simulink model "p4_system_arch_master"  (R2020a)
settings: Solver=VariableStepAuto  StartTime=0.0  StopTime=10.0  RelTol=1e-3
(part 9 of 11)

== system p4_system_arch_master/System 5 : Enclosure and Sealing System X/5.3 Component Enclosure Peripherals X/5.3.1 Fixing, Indexation and Labeling System/5.3.1.1 Gearbox Enclosures Fixing System/5.3.1.1.20 LV connector fixing screws ==
  LV connector fixing screw 1 : ModelReference  ModelNameDialog=M6x12  SimulationMode=Normal  ModelReferenceVersion=1.1
      settings: PortSchema="{\"entries\":[{\"content\":{\"headerSize\":38,\"margin\":15,\"minimumSpacing\":25,\"sides\":[{\"content\":{\"connectorIds\":[]},\"type\":\"ConnectorPlacement.EquallySpacedRectSide\",\"uuid\":\"a1de0a4a-4383-4256-97c8-b4b7017d79c3\"},{\"content\":{\"connectorIds\":[],\"side\":\"RIGHT\"},\"type\":\"ConnectorPlacement.EquallySpacedRectSide\",\"uuid\":\"b959f0e1-b665-4773-a9ab-23b80a79bba3\"},{\"content\":{\"connectorIds\":[],\"side\":\"TOP\"},\"type\":\"ConnectorPlacement.EquallySpacedRectSide\",\"uuid\":\"884e98bd-fa8a-4556-86a7-182eb6de8f96\"}]},\"type\":\"ConnectorPlacement.EquallySpacedConnector\",\"uuid\":\"31d5ce3f-6fbe-45a5-a872-1e90bd0aea01\"}],\"packageUris\":[\"http://schema.mathworks.com/mf0/Connector/19700101\"],\"version\":\"1.0\"}"
  LV connector fixing screw 2 : ModelReference  ModelNameDialog=M6x12  SimulationMode=Normal  ModelReferenceVersion=1.1
      settings: PortSchema="{\"entries\":[{\"content\":{\"headerSize\":38,\"margin\":15,\"minimumSpacing\":25,\"sides\":[{\"content\":{\"connectorIds\":[]},\"type\":\"ConnectorPlacement.EquallySpacedRectSide\",\"uuid\":\"a1de0a4a-4383-4256-97c8-b4b7017d79c3\"},{\"content\":{\"connectorIds\":[],\"side\":\"RIGHT\"},\"type\":\"ConnectorPlacement.EquallySpacedRectSide\",\"uuid\":\"b959f0e1-b665-4773-a9ab-23b80a79bba3\"},{\"content\":{\"connectorIds\":[],\"side\":\"TOP\"},\"type\":\"ConnectorPlacement.EquallySpacedRectSide\",\"uuid\":\"884e98bd-fa8a-4556-86a7-182eb6de8f96\"}]},\"type\":\"ConnectorPlacement.EquallySpacedConnector\",\"uuid\":\"31d5ce3f-6fbe-45a5-a872-1e90bd0aea01\"}],\"packageUris\":[\"http://schema.mathworks.com/mf0/Connector/19700101\"],\"version\":\"1.0\"}"

== system p4_system_arch_master/System 5 : Enclosure and Sealing System X/5.3 Component Enclosure Peripherals X/5.3.1 Fixing, Indexation and Labeling System/5.3.1.1 Gearbox Enclosures Fixing System/5.3.1.1.21 DC connector fixing screws ==
  DC Connector Fixing Screw 1 : Subsystem
      settings: PortSchema="{\"entries\":[{\"content\":{\"headerSize\":26,\"margin\":15,\"minimumSpacing\":25,\"sides\":[{\"content\":{\"connectorIds\":[]},\"type\":\"ConnectorPlacement.EquallySpacedRectSide\",\"uuid\":\"f8ee33a9-954f-44c6-a821-b5353f3278fa\"},{\"content\":{\"connectorIds\":[],\"side\":\"RIGHT\"},\"type\":\"ConnectorPlacement.EquallySpacedRectSide\",\"uuid\":\"385f1e4f-1c89-4afc-9c19-76a078cf90bc\"},{\"content\":{\"connectorIds\":[],\"side\":\"TOP\"},\"type\":\"ConnectorPlacement.EquallySpacedRectSide\",\"uuid\":\"fc91fa49-46f5-4ba7-960e-7bda5e0416d1\"}]},\"type\":\"ConnectorPlacement.EquallySpacedConnector\",\"uuid\":\"4bf08bc6-c7ce-47fb-af04-cd9d2b5f8092\"}],\"packageUris\":[\"http://schema.mathworks.com/mf0/Connector/19700101\"],\"version\":\"1.0\"}"
  DC Connector Fixing Screw 2 : Subsystem
      settings: PortSchema="{\"entries\":[{\"content\":{\"headerSize\":26,\"margin\":15,\"minimumSpacing\":25,\"sides\":[{\"content\":{\"connectorIds\":[]},\"type\":\"ConnectorPlacement.EquallySpacedRectSide\",\"uuid\":\"f8ee33a9-954f-44c6-a821-b5353f3278fa\"},{\"content\":{\"connectorIds\":[],\"side\":\"RIGHT\"},\"type\":\"ConnectorPlacement.EquallySpacedRectSide\",\"uuid\":\"385f1e4f-1c89-4afc-9c19-76a078cf90bc\"},{\"content\":{\"connectorIds\":[],\"side\":\"TOP\"},\"type\":\"ConnectorPlacement.EquallySpacedRectSide\",\"uuid\":\"fc91fa49-46f5-4ba7-960e-7bda5e0416d1\"}]},\"type\":\"ConnectorPlacement.EquallySpacedConnector\",\"uuid\":\"4bf08bc6-c7ce-47fb-af04-cd9d2b5f8092\"}],\"packageUris\":[\"http://schema.mathworks.com/mf0/Connector/19700101\"],\"version\":\"1.0\"}"

== system p4_system_arch_master/System 5 : Enclosure and Sealing System X/5.3 Component Enclosure Peripherals X/5.3.1 Fixing, Indexation and Labeling System/5.3.1.1 Gearbox Enclosures Fixing System/5.3.1.1.25 Breather Labyrinth Cover Bolts ==

== system p4_system_arch_master/System 5 : Enclosure and Sealing System X/5.3 Component Enclosure Peripherals X/5.3.1 Fixing, Indexation and Labeling System/5.3.1.1 Gearbox Enclosures Fixing System/5.3.1.1.5 Shifting Actuator Screws ==

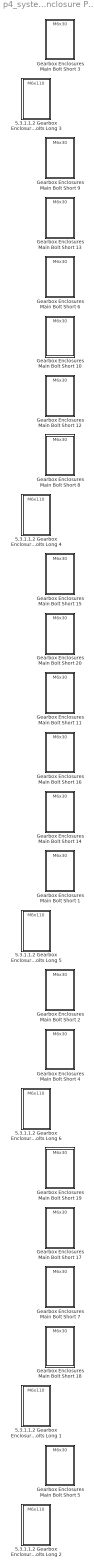
== system p4_system_arch_master/System 5 : Enclosure and Sealing System X/5.3 Component Enclosure Peripherals X/5.3.1 Fixing, Indexation and Labeling System/5.3.1.1 Gearbox Enclosures Fixing System/Gearbox Enclosure Main Bolt System ==
  5.3.1.1.2 Gearbox Enclosures Main Bolts Long {1..6} (6 alike) : ModelReference  ModelNameDialog=M6x110  SimulationMode=Normal  ModelReferenceVersion=1.1
      settings: PortSchema="{\"entries\":[{\"content\":{\"headerSize\":38,\"margin\":15,\"minimumSpacing\":25,\"sides\":[{\"content\":{\"connectorIds\":[]},\"type\":\"ConnectorPlacement.EquallySpacedRectSide\",\"uuid\":\"a1de0a4a-4383-4256-97c8-b4b7017d79c3\"},{\"content\":{\"connectorIds\":[],\"side\":\"RIGHT\"},\"type\":\"ConnectorPlacement.EquallySpacedRectSide\",\"uuid\":\"b959f0e1-b665-4773-a9ab-23b80a79bba3\"},{\"content\":{\"connectorIds\":[],\"side\":\"TOP\"},\"type\":\"ConnectorPlacement.EquallySpacedRectSide\",\"uuid\":\"884e98bd-fa8a-4556-86a7-182eb6de8f96\"}]},\"type\":\"ConnectorPlacement.EquallySpacedConnector\",\"uuid\":\"31d5ce3f-6fbe-45a5-a872-1e90bd0aea01\"}],\"packageUris\":[\"http://schema.mathworks.com/mf0/Connector/19700101\"],\"version\":\"1.0\"}"
  Gearbox Enclosures Main Bolt Short {1..20} (20 alike) : ModelReference  ModelNameDialog=M6x30  SimulationMode=Normal  ModelReferenceVersion=1.1
      settings: PortSchema="{\"entries\":[{\"content\":{\"headerSize\":38,\"margin\":15,\"minimumSpacing\":25,\"sides\":[{\"content\":{\"connectorIds\":[]},\"type\":\"ConnectorPlacement.EquallySpacedRectSide\",\"uuid\":\"a1de0a4a-4383-4256-97c8-b4b7017d79c3\"},{\"content\":{\"connectorIds\":[],\"side\":\"RIGHT\"},\"type\":\"ConnectorPlacement.EquallySpacedRectSide\",\"uuid\":\"b959f0e1-b665-4773-a9ab-23b80a79bba3\"},{\"content\":{\"connectorIds\":[],\"side\":\"TOP\"},\"type\":\"ConnectorPlacement.EquallySpacedRectSide\",\"uuid\":\"884e98bd-fa8a-4556-86a7-182eb6de8f96\"}]},\"type\":\"ConnectorPlacement.EquallySpacedConnector\",\"uuid\":\"31d5ce3f-6fbe-45a5-a872-1e90bd0aea01\"}],\"packageUris\":[\"http://schema.mathworks.com/mf0/Connector/19700101\"],\"version\":\"1.0\"}"

== system p4_system_arch_master/System 5 : Enclosure and Sealing System X/5.3 Component Enclosure Peripherals X/5.3.1 Fixing, Indexation and Labeling System/5.3.1.1 Gearbox Enclosures Fixing System/I//O Module Bolt System ==

== system p4_system_arch_master/System 5 : Enclosure and Sealing System X/5.3 Component Enclosure Peripherals X/5.3.1 Fixing, Indexation and Labeling System/5.3.1.1 Gearbox Enclosures Fixing System/Inverter fixing screws System ==
  5.3.1.1.16 Top inverter cover fixing screws : Subsystem
      settings: PortSchema="{\"entries\":[{\"content\":{\"headerSize\":26,\"margin\":15,\"minimumSpacing\":25,\"sides\":[{\"content\":{\"connectorIds\":[]},\"type\":\"ConnectorPlacement.EquallySpacedRectSide\",\"uuid\":\"f8ee33a9-954f-44c6-a821-b5353f3278fa\"},{\"content\":{\"connectorIds\":[],\"side\":\"RIGHT\"},\"type\":\"ConnectorPlacement.EquallySpacedRectSide\",\"uuid\":\"385f1e4f-1c89-4afc-9c19-76a078cf90bc\"},{\"content\":{\"connectorIds\":[],\"side\":\"TOP\"},\"type\":\"ConnectorPlacement.EquallySpacedRectSide\",\"uuid\":\"fc91fa49-46f5-4ba7-960e-7bda5e0416d1\"}]},\"type\":\"ConnectorPlacement.EquallySpacedConnector\",\"uuid\":\"4bf08bc6-c7ce-47fb-af04-cd9d2b5f8092\"}],\"packageUris\":[\"http://schema.mathworks.com/mf0/Connector/19700101\"],\"version\":\"1.0\"}"
  5.3.1.1.17 Inverter fixing screws : Subsystem
      settings: PortSchema="{\"entries\":[{\"content\":{\"headerSize\":26,\"margin\":15,\"minimumSpacing\":25,\"sides\":[{\"content\":{\"connectorIds\":[]},\"type\":\"ConnectorPlacement.EquallySpacedRectSide\",\"uuid\":\"f8ee33a9-954f-44c6-a821-b5353f3278fa\"},{\"content\":{\"connectorIds\":[],\"side\":\"RIGHT\"},\"type\":\"ConnectorPlacement.EquallySpacedRectSide\",\"uuid\":\"385f1e4f-1c89-4afc-9c19-76a078cf90bc\"},{\"content\":{\"connectorIds\":[],\"side\":\"TOP\"},\"type\":\"ConnectorPlacement.EquallySpacedRectSide\",\"uuid\":\"fc91fa49-46f5-4ba7-960e-7bda5e0416d1\"}]},\"type\":\"ConnectorPlacement.EquallySpacedConnector\",\"uuid\":\"4bf08bc6-c7ce-47fb-af04-cd9d2b5f8092\"}],\"packageUris\":[\"http://schema.mathworks.com/mf0/Connector/19700101\"],\"version\":\"1.0\"}"

== system p4_system_arch_master/System 5 : Enclosure and Sealing System X/5.3 Component Enclosure Peripherals X/5.3.1 Fixing, Indexation and Labeling System/5.3.1.1 Gearbox Enclosures Fixing System/Motorcover Securing System ==
  5.3.1.1.12 Motor cover fixing screws short : Subsystem
      settings: PortSchema="{\"entries\":[{\"content\":{\"headerSize\":26,\"margin\":15,\"minimumSpacing\":25,\"sides\":[{\"content\":{\"connectorIds\":[]},\"type\":\"ConnectorPlacement.EquallySpacedRectSide\",\"uuid\":\"f8ee33a9-954f-44c6-a821-b5353f3278fa\"},{\"content\":{\"connectorIds\":[],\"side\":\"RIGHT\"},\"type\":\"ConnectorPlacement.EquallySpacedRectSide\",\"uuid\":\"385f1e4f-1c89-4afc-9c19-76a078cf90bc\"},{\"content\":{\"connectorIds\":[],\"side\":\"TOP\"},\"type\":\"ConnectorPlacement.EquallySpacedRectSide\",\"uuid\":\"fc91fa49-46f5-4ba7-960e-7bda5e0416d1\"}]},\"type\":\"ConnectorPlacement.EquallySpacedConnector\",\"uuid\":\"4bf08bc6-c7ce-47fb-af04-cd9d2b5f8092\"}],\"packageUris\":[\"http://schema.mathworks.com/mf0/Connector/19700101\"],\"version\":\"1.0\"}"
  5.3.1.1.13 Motor cover fixing screws long : Subsystem
      settings: PortSchema="{\"entries\":[{\"content\":{\"headerSize\":26,\"margin\":15,\"minimumSpacing\":25,\"sides\":[{\"content\":{\"connectorIds\":[]},\"type\":\"ConnectorPlacement.EquallySpacedRectSide\",\"uuid\":\"f8ee33a9-954f-44c6-a821-b5353f3278fa\"},{\"content\":{\"connectorIds\":[],\"side\":\"RIGHT\"},\"type\":\"ConnectorPlacement.EquallySpacedRectSide\",\"uuid\":\"385f1e4f-1c89-4afc-9c19-76a078cf90bc\"},{\"content\":{\"connectorIds\":[],\"side\":\"TOP\"},\"type\":\"ConnectorPlacement.EquallySpacedRectSide\",\"uuid\":\"fc91fa49-46f5-4ba7-960e-7bda5e0416d1\"}]},\"type\":\"ConnectorPlacement.EquallySpacedConnector\",\"uuid\":\"4bf08bc6-c7ce-47fb-af04-cd9d2b5f8092\"}],\"packageUris\":[\"http://schema.mathworks.com/mf0/Connector/19700101\"],\"version\":\"1.0\"}"

== system p4_system_arch_master/System 5 : Enclosure and Sealing System X/5.3 Component Enclosure Peripherals X/5.3.1 Fixing, Indexation and Labeling System/5.3.1.1 Gearbox Enclosures Fixing System/Oil Baffle securing System ==
  5.3.1.1.19 Oil baffle RH bolts : Subsystem
      settings: PortSchema="{\"entries\":[{\"content\":{\"headerSize\":26,\"margin\":15,\"minimumSpacing\":25,\"sides\":[{\"content\":{\"connectorIds\":[]},\"type\":\"ConnectorPlacement.EquallySpacedRectSide\",\"uuid\":\"f8ee33a9-954f-44c6-a821-b5353f3278fa\"},{\"content\":{\"connectorIds\":[],\"side\":\"RIGHT\"},\"type\":\"ConnectorPlacement.EquallySpacedRectSide\",\"uuid\":\"385f1e4f-1c89-4afc-9c19-76a078cf90bc\"},{\"content\":{\"connectorIds\":[],\"side\":\"TOP\"},\"type\":\"ConnectorPlacement.EquallySpacedRectSide\",\"uuid\":\"fc91fa49-46f5-4ba7-960e-7bda5e0416d1\"}]},\"type\":\"ConnectorPlacement.EquallySpacedConnector\",\"uuid\":\"4bf08bc6-c7ce-47fb-af04-cd9d2b5f8092\"}],\"packageUris\":[\"http://schema.mathworks.com/mf0/Connector/19700101\"],\"version\":\"1.0\"}"
  "5.3.1.1.9 Rear Oil Baffle LH Bolts " : Subsystem
      settings: PortSchema="{\"entries\":[{\"content\":{\"headerSize\":26,\"margin\":15,\"minimumSpacing\":25,\"sides\":[{\"content\":{\"connectorIds\":[]},\"type\":\"ConnectorPlacement.EquallySpacedRectSide\",\"uuid\":\"f8ee33a9-954f-44c6-a821-b5353f3278fa\"},{\"content\":{\"connectorIds\":[],\"side\":\"RIGHT\"},\"type\":\"ConnectorPlacement.EquallySpacedRectSide\",\"uuid\":\"385f1e4f-1c89-4afc-9c19-76a078cf90bc\"},{\"content\":{\"connectorIds\":[],\"side\":\"TOP\"},\"type\":\"ConnectorPlacement.EquallySpacedRectSide\",\"uuid\":\"fc91fa49-46f5-4ba7-960e-7bda5e0416d1\"}]},\"type\":\"ConnectorPlacement.EquallySpacedConnector\",\"uuid\":\"4bf08bc6-c7ce-47fb-af04-cd9d2b5f8092\"}],\"packageUris\":[\"http://schema.mathworks.com/mf0/Connector/19700101\"],\"version\":\"1.0\"}"

== system p4_system_arch_master/System 5 : Enclosure and Sealing System X/5.3 Component Enclosure Peripherals X/5.3.1 Fixing, Indexation and Labeling System/5.3.1.1 Gearbox Enclosures Fixing System/Oil Catcher Bolts System ==
  5.3.1.1.7 Oil Catcher B3 Bolts : Subsystem
      settings: PortSchema="{\"entries\":[{\"content\":{\"headerSize\":26,\"margin\":15,\"minimumSpacing\":25,\"sides\":[{\"content\":{\"connectorIds\":[]},\"type\":\"ConnectorPlacement.EquallySpacedRectSide\",\"uuid\":\"f8ee33a9-954f-44c6-a821-b5353f3278fa\"},{\"content\":{\"connectorIds\":[],\"side\":\"RIGHT\"},\"type\":\"ConnectorPlacement.EquallySpacedRectSide\",\"uuid\":\"385f1e4f-1c89-4afc-9c19-76a078cf90bc\"},{\"content\":{\"connectorIds\":[],\"side\":\"TOP\"},\"type\":\"ConnectorPlacement.EquallySpacedRectSide\",\"uuid\":\"fc91fa49-46f5-4ba7-960e-7bda5e0416d1\"}]},\"type\":\"ConnectorPlacement.EquallySpacedConnector\",\"uuid\":\"4bf08bc6-c7ce-47fb-af04-cd9d2b5f8092\"}],\"packageUris\":[\"http://schema.mathworks.com/mf0/Connector/19700101\"],\"version\":\"1.0\"}"
  5.3.1.1.8 Oil Catcher B1 Bolts : Subsystem
      settings: PortSchema="{\"entries\":[{\"content\":{\"headerSize\":26,\"margin\":15,\"minimumSpacing\":25,\"sides\":[{\"content\":{\"connectorIds\":[]},\"type\":\"ConnectorPlacement.EquallySpacedRectSide\",\"uuid\":\"f8ee33a9-954f-44c6-a821-b5353f3278fa\"},{\"content\":{\"connectorIds\":[],\"side\":\"RIGHT\"},\"type\":\"ConnectorPlacement.EquallySpacedRectSide\",\"uuid\":\"385f1e4f-1c89-4afc-9c19-76a078cf90bc\"},{\"content\":{\"connectorIds\":[],\"side\":\"TOP\"},\"type\":\"ConnectorPlacement.EquallySpacedRectSide\",\"uuid\":\"fc91fa49-46f5-4ba7-960e-7bda5e0416d1\"}]},\"type\":\"ConnectorPlacement.EquallySpacedConnector\",\"uuid\":\"4bf08bc6-c7ce-47fb-af04-cd9d2b5f8092\"}],\"packageUris\":[\"http://schema.mathworks.com/mf0/Connector/19700101\"],\"version\":\"1.0\"}"

== system p4_system_arch_master/System 5 : Enclosure and Sealing System X/5.3 Component Enclosure Peripherals X/5.3.1 Fixing, Indexation and Labeling System/5.3.1.1 Gearbox Enclosures Fixing System/Resolver System ==
  5.3.1.1.14 Resolver fixing screws : Subsystem
      settings: PortSchema="{\"entries\":[{\"content\":{\"headerSize\":26,\"margin\":15,\"minimumSpacing\":25,\"sides\":[{\"content\":{\"connectorIds\":[]},\"type\":\"ConnectorPlacement.EquallySpacedRectSide\",\"uuid\":\"f8ee33a9-954f-44c6-a821-b5353f3278fa\"},{\"content\":{\"connectorIds\":[],\"side\":\"RIGHT\"},\"type\":\"ConnectorPlacement.EquallySpacedRectSide\",\"uuid\":\"385f1e4f-1c89-4afc-9c19-76a078cf90bc\"},{\"content\":{\"connectorIds\":[],\"side\":\"TOP\"},\"type\":\"ConnectorPlacement.EquallySpacedRectSide\",\"uuid\":\"fc91fa49-46f5-4ba7-960e-7bda5e0416d1\"}]},\"type\":\"ConnectorPlacement.EquallySpacedConnector\",\"uuid\":\"4bf08bc6-c7ce-47fb-af04-cd9d2b5f8092\"}],\"packageUris\":[\"http://schema.mathworks.com/mf0/Connector/19700101\"],\"version\":\"1.0\"}"
  5.3.1.1.15 Resolver cover fixing screws : Subsystem
      settings: PortSchema="{\"entries\":[{\"content\":{\"headerSize\":26,\"margin\":15,\"minimumSpacing\":25,\"sides\":[{\"content\":{\"connectorIds\":[]},\"type\":\"ConnectorPlacement.EquallySpacedRectSide\",\"uuid\":\"f8ee33a9-954f-44c6-a821-b5353f3278fa\"},{\"content\":{\"connectorIds\":[],\"side\":\"RIGHT\"},\"type\":\"ConnectorPlacement.EquallySpacedRectSide\",\"uuid\":\"385f1e4f-1c89-4afc-9c19-76a078cf90bc\"},{\"content\":{\"connectorIds\":[],\"side\":\"TOP\"},\"type\":\"ConnectorPlacement.EquallySpacedRectSide\",\"uuid\":\"fc91fa49-46f5-4ba7-960e-7bda5e0416d1\"}]},\"type\":\"ConnectorPlacement.EquallySpacedConnector\",\"uuid\":\"4bf08bc6-c7ce-47fb-af04-cd9d2b5f8092\"}],\"packageUris\":[\"http://schema.mathworks.com/mf0/Connector/19700101\"],\"version\":\"1.0\"}"
  5.3.1.1.24 Resolver Plate : Subsystem
      settings: PortSchema="{\"entries\":[{\"content\":{\"headerSize\":26,\"margin\":15,\"minimumSpacing\":25,\"sides\":[{\"content\":{\"connectorIds\":[]},\"type\":\"ConnectorPlacement.EquallySpacedRectSide\",\"uuid\":\"f8ee33a9-954f-44c6-a821-b5353f3278fa\"},{\"content\":{\"connectorIds\":[],\"side\":\"RIGHT\"},\"type\":\"ConnectorPlacement.EquallySpacedRectSide\",\"uuid\":\"385f1e4f-1c89-4afc-9c19-76a078cf90bc\"},{\"content\":{\"connectorIds\":[],\"side\":\"TOP\"},\"type\":\"ConnectorPlacement.EquallySpacedRectSide\",\"uuid\":\"fc91fa49-46f5-4ba7-960e-7bda5e0416d1\"}]},\"type\":\"ConnectorPlacement.EquallySpacedConnector\",\"uuid\":\"4bf08bc6-c7ce-47fb-af04-cd9d2b5f8092\"}],\"packageUris\":[\"http://schema.mathworks.com/mf0/Connector/19700101\"],\"version\":\"1.0\"}"

== system p4_system_arch_master/System 5 : Enclosure and Sealing System X/5.3 Component Enclosure Peripherals X/5.3.1 Fixing, Indexation and Labeling System/5.3.1.1 Gearbox Enclosures Fixing System/Shifting Angle Sensor Bolts System ==
  5.3.1.1.23 Shifting Angle Sensor Bolts : Subsystem
      settings: PortSchema="{\"entries\":[{\"content\":{\"headerSize\":26,\"margin\":15,\"minimumSpacing\":25,\"sides\":[{\"content\":{\"connectorIds\":[]},\"type\":\"ConnectorPlacement.EquallySpacedRectSide\",\"uuid\":\"f8ee33a9-954f-44c6-a821-b5353f3278fa\"},{\"content\":{\"connectorIds\":[],\"side\":\"RIGHT\"},\"type\":\"ConnectorPlacement.EquallySpacedRectSide\",\"uuid\":\"385f1e4f-1c89-4afc-9c19-76a078cf90bc\"},{\"content\":{\"connectorIds\":[],\"side\":\"TOP\"},\"type\":\"ConnectorPlacement.EquallySpacedRectSide\",\"uuid\":\"fc91fa49-46f5-4ba7-960e-7bda5e0416d1\"}]},\"type\":\"ConnectorPlacement.EquallySpacedConnector\",\"uuid\":\"4bf08bc6-c7ce-47fb-af04-cd9d2b5f8092\"}],\"packageUris\":[\"http://schema.mathworks.com/mf0/Connector/19700101\"],\"version\":\"1.0\"}"

== system p4_system_arch_master/System 5 : Enclosure and Sealing System X/5.3 Component Enclosure Peripherals X/5.3.1 Fixing, Indexation and Labeling System/5.3.1.1 Gearbox Enclosures Fixing System/Shifting Cover Bolts System ==
  5.3.1.1.4 Shifting Cover Bolt 1 : Subsystem
      settings: PortSchema="{\"entries\":[{\"content\":{\"headerSize\":26,\"margin\":15,\"minimumSpacing\":25,\"sides\":[{\"content\":{\"connectorIds\":[]},\"type\":\"ConnectorPlacement.EquallySpacedRectSide\",\"uuid\":\"f8ee33a9-954f-44c6-a821-b5353f3278fa\"},{\"content\":{\"connectorIds\":[],\"side\":\"RIGHT\"},\"type\":\"ConnectorPlacement.EquallySpacedRectSide\",\"uuid\":\"385f1e4f-1c89-4afc-9c19-76a078cf90bc\"},{\"content\":{\"connectorIds\":[],\"side\":\"TOP\"},\"type\":\"ConnectorPlacement.EquallySpacedRectSide\",\"uuid\":\"fc91fa49-46f5-4ba7-960e-7bda5e0416d1\"}]},\"type\":\"ConnectorPlacement.EquallySpacedConnector\",\"uuid\":\"4bf08bc6-c7ce-47fb-af04-cd9d2b5f8092\"}],\"packageUris\":[\"http://schema.mathworks.com/mf0/Connector/19700101\"],\"version\":\"1.0\"}"
  5.3.1.1.4 Shifting Cover Bolt 2 : Subsystem
      settings: PortSchema="{\"entries\":[{\"content\":{\"headerSize\":26,\"margin\":15,\"minimumSpacing\":25,\"sides\":[{\"content\":{\"connectorIds\":[]},\"type\":\"ConnectorPlacement.EquallySpacedRectSide\",\"uuid\":\"f8ee33a9-954f-44c6-a821-b5353f3278fa\"},{\"content\":{\"connectorIds\":[],\"side\":\"RIGHT\"},\"type\":\"ConnectorPlacement.EquallySpacedRectSide\",\"uuid\":\"385f1e4f-1c89-4afc-9c19-76a078cf90bc\"},{\"content\":{\"connectorIds\":[],\"side\":\"TOP\"},\"type\":\"ConnectorPlacement.EquallySpacedRectSide\",\"uuid\":\"fc91fa49-46f5-4ba7-960e-7bda5e0416d1\"}]},\"type\":\"ConnectorPlacement.EquallySpacedConnector\",\"uuid\":\"4bf08bc6-c7ce-47fb-af04-cd9d2b5f8092\"}],\"packageUris\":[\"http://schema.mathworks.com/mf0/Connector/19700101\"],\"version\":\"1.0\"}"
  5.3.1.1.4 Shifting Cover Bolt 3 : Subsystem
      settings: PortSchema="{\"entries\":[{\"content\":{\"headerSize\":26,\"margin\":15,\"minimumSpacing\":25,\"sides\":[{\"content\":{\"connectorIds\":[]},\"type\":\"ConnectorPlacement.EquallySpacedRectSide\",\"uuid\":\"f8ee33a9-954f-44c6-a821-b5353f3278fa\"},{\"content\":{\"connectorIds\":[],\"side\":\"RIGHT\"},\"type\":\"ConnectorPlacement.EquallySpacedRectSide\",\"uuid\":\"385f1e4f-1c89-4afc-9c19-76a078cf90bc\"},{\"content\":{\"connectorIds\":[],\"side\":\"TOP\"},\"type\":\"ConnectorPlacement.EquallySpacedRectSide\",\"uuid\":\"fc91fa49-46f5-4ba7-960e-7bda5e0416d1\"}]},\"type\":\"ConnectorPlacement.EquallySpacedConnector\",\"uuid\":\"4bf08bc6-c7ce-47fb-af04-cd9d2b5f8092\"}],\"packageUris\":[\"http://schema.mathworks.com/mf0/Connector/19700101\"],\"version\":\"1.0\"}"
  5.3.1.1.4 Shifting Cover Bolt 4 : Subsystem
      settings: PortSchema="{\"entries\":[{\"content\":{\"headerSize\":26,\"margin\":15,\"minimumSpacing\":25,\"sides\":[{\"content\":{\"connectorIds\":[]},\"type\":\"ConnectorPlacement.EquallySpacedRectSide\",\"uuid\":\"f8ee33a9-954f-44c6-a821-b5353f3278fa\"},{\"content\":{\"connectorIds\":[],\"side\":\"RIGHT\"},\"type\":\"ConnectorPlacement.EquallySpacedRectSide\",\"uuid\":\"385f1e4f-1c89-4afc-9c19-76a078cf90bc\"},{\"content\":{\"connectorIds\":[],\"side\":\"TOP\"},\"type\":\"ConnectorPlacement.EquallySpacedRectSide\",\"uuid\":\"fc91fa49-46f5-4ba7-960e-7bda5e0416d1\"}]},\"type\":\"ConnectorPlacement.EquallySpacedConnector\",\"uuid\":\"4bf08bc6-c7ce-47fb-af04-cd9d2b5f8092\"}],\"packageUris\":[\"http://schema.mathworks.com/mf0/Connector/19700101\"],\"version\":\"1.0\"}"

== system p4_system_arch_master/System 5 : Enclosure and Sealing System X/5.3 Component Enclosure Peripherals X/5.3.1 Fixing, Indexation and Labeling System/5.3.1.1 Gearbox Enclosures Fixing System/Speed Sensor Bolt System ==
  5.3.1.1.6 Speed Sensor LH Bolt : ModelReference  ModelNameDialog=M6x14  SimulationMode=Normal  ModelReferenceVersion=1.1
      settings: PortSchema="{\"entries\":[{\"content\":{\"headerSize\":38,\"margin\":15,\"minimumSpacing\":25,\"sides\":[{\"content\":{\"connectorIds\":[]},\"type\":\"ConnectorPlacement.EquallySpacedRectSide\",\"uuid\":\"a1de0a4a-4383-4256-97c8-b4b7017d79c3\"},{\"content\":{\"connectorIds\":[],\"side\":\"RIGHT\"},\"type\":\"ConnectorPlacement.EquallySpacedRectSide\",\"uuid\":\"b959f0e1-b665-4773-a9ab-23b80a79bba3\"},{\"content\":{\"connectorIds\":[],\"side\":\"TOP\"},\"type\":\"ConnectorPlacement.EquallySpacedRectSide\",\"uuid\":\"884e98bd-fa8a-4556-86a7-182eb6de8f96\"}]},\"type\":\"ConnectorPlacement.EquallySpacedConnector\",\"uuid\":\"31d5ce3f-6fbe-45a5-a872-1e90bd0aea01\"}],\"packageUris\":[\"http://schema.mathworks.com/mf0/Connector/19700101\"],\"version\":\"1.0\"}"
  5.3.1.1.6 Speed Sensor RH Bolt : ModelReference  ModelNameDialog=M6x14  SimulationMode=Normal  ModelReferenceVersion=1.1
      settings: PortSchema="{\"entries\":[{\"content\":{\"headerSize\":38,\"margin\":15,\"minimumSpacing\":25,\"sides\":[{\"content\":{\"connectorIds\":[]},\"type\":\"ConnectorPlacement.EquallySpacedRectSide\",\"uuid\":\"a1de0a4a-4383-4256-97c8-b4b7017d79c3\"},{\"content\":{\"connectorIds\":[],\"side\":\"RIGHT\"},\"type\":\"ConnectorPlacement.EquallySpacedRectSide\",\"uuid\":\"b959f0e1-b665-4773-a9ab-23b80a79bba3\"},{\"content\":{\"connectorIds\":[],\"side\":\"TOP\"},\"type\":\"ConnectorPlacement.EquallySpacedRectSide\",\"uuid\":\"884e98bd-fa8a-4556-86a7-182eb6de8f96\"}]},\"type\":\"ConnectorPlacement.EquallySpacedConnector\",\"uuid\":\"31d5ce3f-6fbe-45a5-a872-1e90bd0aea01\"}],\"packageUris\":[\"http://schema.mathworks.com/mf0/Connector/19700101\"],\"version\":\"1.0\"}"

== system p4_system_arch_master/System 5 : Enclosure and Sealing System X/5.3 Component Enclosure Peripherals X/5.3.1 Fixing, Indexation and Labeling System/5.3.1.1 Gearbox Enclosures Fixing System/Stator Securing System ==
  5.3.1.1.10 Stator bolt {1..4} (4 alike) : ModelReference  ModelNameDialog=M8x220  SimulationMode=Normal  ModelReferenceVersion=1.1
      settings: PortSchema="{\"entries\":[{\"content\":{\"headerSize\":38,\"margin\":15,\"minimumSpacing\":25,\"sides\":[{\"content\":{\"connectorIds\":[]},\"type\":\"ConnectorPlacement.EquallySpacedRectSide\",\"uuid\":\"a1de0a4a-4383-4256-97c8-b4b7017d79c3\"},{\"content\":{\"connectorIds\":[],\"side\":\"RIGHT\"},\"type\":\"ConnectorPlacement.EquallySpacedRectSide\",\"uuid\":\"b959f0e1-b665-4773-a9ab-23b80a79bba3\"},{\"content\":{\"connectorIds\":[],\"side\":\"TOP\"},\"type\":\"ConnectorPlacement.EquallySpacedRectSide\",\"uuid\":\"884e98bd-fa8a-4556-86a7-182eb6de8f96\"}]},\"type\":\"ConnectorPlacement.EquallySpacedConnector\",\"uuid\":\"31d5ce3f-6fbe-45a5-a872-1e90bd0aea01\"}],\"packageUris\":[\"http://schema.mathworks.com/mf0/Connector/19700101\"],\"version\":\"1.0\"}"
  5.3.1.1.11 Stator piston bush (sleeves) {1..4} (4 alike) : ModelReference  ModelNameDialog=StatorPistonBushSleeves  SimulationMode=Normal  ModelReferenceVersion=1.2
      settings: PortSchema="{\"entries\":[{\"content\":{\"headerSize\":38,\"margin\":15,\"minimumSpacing\":25,\"sides\":[{\"content\":{\"connectorIds\":[]},\"type\":\"ConnectorPlacement.EquallySpacedRectSide\",\"uuid\":\"a1de0a4a-4383-4256-97c8-b4b7017d79c3\"},{\"content\":{\"connectorIds\":[],\"side\":\"RIGHT\"},\"type\":\"ConnectorPlacement.EquallySpacedRectSide\",\"uuid\":\"b959f0e1-b665-4773-a9ab-23b80a79bba3\"},{\"content\":{\"connectorIds\":[],\"side\":\"TOP\"},\"type\":\"ConnectorPlacement.EquallySpacedRectSide\",\"uuid\":\"884e98bd-fa8a-4556-86a7-182eb6de8f96\"}]},\"type\":\"ConnectorPlacement.EquallySpacedConnector\",\"uuid\":\"31d5ce3f-6fbe-45a5-a872-1e90bd0aea01\"}],\"packageUris\":[\"http://schema.mathworks.com/mf0/Connector/19700101\"],\"version\":\"1.0\"}"

== system p4_system_arch_master/System 5 : Enclosure and Sealing System X/5.3 Component Enclosure Peripherals X/5.3.2 Lubrication and Cooling Peripherals/5.3.2.1 Lubrication System Peripherals/5.3.2.1.1 Oil filling plug ==

== system p4_system_arch_master/System 5 : Enclosure and Sealing System X/5.3 Component Enclosure Peripherals X/5.3.2 Lubrication and Cooling Peripherals/5.3.2.1 Lubrication System Peripherals/5.3.2.1.2 Oil Catcher B1 ==

== system p4_system_arch_master/System 5 : Enclosure and Sealing System X/5.3 Component Enclosure Peripherals X/5.3.2 Lubrication and Cooling Peripherals/5.3.2.1 Lubrication System Peripherals/5.3.2.1.3 Oil Catcher B3 ==

== system p4_system_arch_master/System 5 : Enclosure and Sealing System X/5.3 Component Enclosure Peripherals X/5.3.2 Lubrication and Cooling Peripherals/5.3.2.1 Lubrication System Peripherals/5.3.2.1.4 Rear Oil Baffle LH ==

== system p4_system_arch_master/System 5 : Enclosure and Sealing System X/5.3 Component Enclosure Peripherals X/5.3.2 Lubrication and Cooling Peripherals/5.3.2.1 Lubrication System Peripherals/5.3.2.1.5 Oil drain plug ==

== system p4_system_arch_master/System 5 : Enclosure and Sealing System X/5.3 Component Enclosure Peripherals X/5.3.2 Lubrication and Cooling Peripherals/5.3.2.1 Lubrication System Peripherals/5.3.2.1.6 Rear Oil Baffle RH ==

== system p4_system_arch_master/System 5 : Enclosure and Sealing System X/5.3 Component Enclosure Peripherals X/5.3.2 Lubrication and Cooling Peripherals/5.3.2.1 Lubrication System Peripherals/5.3.2.1.7 Breather Labyrinth Cover ==

== system p4_system_arch_master/System 5 : Enclosure and Sealing System X/5.3 Component Enclosure Peripherals X/5.3.2 Lubrication and Cooling Peripherals/5.3.2.1 Lubrication System Peripherals/5.3.2.1.8 Oil Disc B3 ==

== system p4_system_arch_master/System 5 : Enclosure and Sealing System X/5.3 Component Enclosure Peripherals X/5.3.2 Lubrication and Cooling Peripherals/5.3.2.3 Gearbox Venting & Aerating System/5.3.2.3.1 Breather ==

== system p4_system_arch_master/System 6 : Sensor and Actuation System/6.1 Sensor System /6.1.4 Gear Selection Position Measurement SubSystem /6.1.4.1 Drum Angular Position Measurement Sensor SubSystem /6.1.4.1.1 Drum Angular Position measurement sensor subsystem - body  ==

== system p4_system_arch_master/System 6 : Sensor and Actuation System/6.1 Sensor System /6.1.4 Gear Selection Position Measurement SubSystem /6.1.4.1 Drum Angular Position Measurement Sensor SubSystem /6.1.4.1.2 Drum Angular Position Measurement Sensor Wires  ==
  Wire 1 : Subsystem
      settings: PortSchema="{\"entries\":[{\"content\":{\"headerSize\":26,\"margin\":15,\"minimumSpacing\":25,\"sides\":[{\"content\":{\"connectorIds\":[]},\"type\":\"ConnectorPlacement.EquallySpacedRectSide\",\"uuid\":\"f8ee33a9-954f-44c6-a821-b5353f3278fa\"},{\"content\":{\"connectorIds\":[],\"side\":\"RIGHT\"},\"type\":\"ConnectorPlacement.EquallySpacedRectSide\",\"uuid\":\"385f1e4f-1c89-4afc-9c19-76a078cf90bc\"},{\"content\":{\"connectorIds\":[],\"side\":\"TOP\"},\"type\":\"ConnectorPlacement.EquallySpacedRectSide\",\"uuid\":\"fc91fa49-46f5-4ba7-960e-7bda5e0416d1\"}]},\"type\":\"ConnectorPlacement.EquallySpacedConnector\",\"uuid\":\"4bf08bc6-c7ce-47fb-af04-cd9d2b5f8092\"}],\"packageUris\":[\"http://schema.mathworks.com/mf0/Connector/19700101\"],\"version\":\"1.0\"}"
  Wire 2 : Subsystem
      settings: PortSchema="{\"entries\":[{\"content\":{\"headerSize\":26,\"margin\":15,\"minimumSpacing\":25,\"sides\":[{\"content\":{\"connectorIds\":[]},\"type\":\"ConnectorPlacement.EquallySpacedRectSide\",\"uuid\":\"f8ee33a9-954f-44c6-a821-b5353f3278fa\"},{\"content\":{\"connectorIds\":[],\"side\":\"RIGHT\"},\"type\":\"ConnectorPlacement.EquallySpacedRectSide\",\"uuid\":\"385f1e4f-1c89-4afc-9c19-76a078cf90bc\"},{\"content\":{\"connectorIds\":[],\"side\":\"TOP\"},\"type\":\"ConnectorPlacement.EquallySpacedRectSide\",\"uuid\":\"fc91fa49-46f5-4ba7-960e-7bda5e0416d1\"}]},\"type\":\"ConnectorPlacement.EquallySpacedConnector\",\"uuid\":\"4bf08bc6-c7ce-47fb-af04-cd9d2b5f8092\"}],\"packageUris\":[\"http://schema.mathworks.com/mf0/Connector/19700101\"],\"version\":\"1.0\"}"
  Wire 3 : Subsystem
      settings: PortSchema="{\"entries\":[{\"content\":{\"headerSize\":26,\"margin\":15,\"minimumSpacing\":25,\"sides\":[{\"content\":{\"connectorIds\":[]},\"type\":\"ConnectorPlacement.EquallySpacedRectSide\",\"uuid\":\"f8ee33a9-954f-44c6-a821-b5353f3278fa\"},{\"content\":{\"connectorIds\":[],\"side\":\"RIGHT\"},\"type\":\"ConnectorPlacement.EquallySpacedRectSide\",\"uuid\":\"385f1e4f-1c89-4afc-9c19-76a078cf90bc\"},{\"content\":{\"connectorIds\":[],\"side\":\"TOP\"},\"type\":\"ConnectorPlacement.EquallySpacedRectSide\",\"uuid\":\"fc91fa49-46f5-4ba7-960e-7bda5e0416d1\"}]},\"type\":\"ConnectorPlacement.EquallySpacedConnector\",\"uuid\":\"4bf08bc6-c7ce-47fb-af04-cd9d2b5f8092\"}],\"packageUris\":[\"http://schema.mathworks.com/mf0/Connector/19700101\"],\"version\":\"1.0\"}"
  Wire 4 : Subsystem
      settings: PortSchema="{\"entries\":[{\"content\":{\"headerSize\":26,\"margin\":15,\"minimumSpacing\":25,\"sides\":[{\"content\":{\"connectorIds\":[]},\"type\":\"ConnectorPlacement.EquallySpacedRectSide\",\"uuid\":\"f8ee33a9-954f-44c6-a821-b5353f3278fa\"},{\"content\":{\"connectorIds\":[],\"side\":\"RIGHT\"},\"type\":\"ConnectorPlacement.EquallySpacedRectSide\",\"uuid\":\"385f1e4f-1c89-4afc-9c19-76a078cf90bc\"},{\"content\":{\"connectorIds\":[],\"side\":\"TOP\"},\"type\":\"ConnectorPlacement.EquallySpacedRectSide\",\"uuid\":\"fc91fa49-46f5-4ba7-960e-7bda5e0416d1\"}]},\"type\":\"ConnectorPlacement.EquallySpacedConnector\",\"uuid\":\"4bf08bc6-c7ce-47fb-af04-cd9d2b5f8092\"}],\"packageUris\":[\"http://schema.mathworks.com/mf0/Connector/19700101\"],\"version\":\"1.0\"}"

== system p4_system_arch_master/System 6 : Sensor and Actuation System/6.1 Sensor System /6.1.4 Gear Selection Position Measurement SubSystem /6.1.4.2 Drum Angular Position Measurement Magnet SubSystem /6.1.4.2.1 Drum Angular position Measurement magent subsystem - body  ==

== system p4_system_arch_master/System 6 : Sensor and Actuation System/6.1 Sensor System /6.1.7 Motor Position Measurement Subsystem /6.1.7.1 Motor Resolver - Stator Subsystem /6.1.7.1.1 Motor Resolver Stator Subsystem - Body ==

== system p4_system_arch_master/System 6 : Sensor and Actuation System/6.1 Sensor System /6.1.7 Motor Position Measurement Subsystem /6.1.7.1 Motor Resolver - Stator Subsystem /6.1.7.1.2 Motor Resolver Stator Subsystem Wires ==
  Wire 1 : Subsystem
      settings: PortSchema="{\"entries\":[{\"content\":{\"headerSize\":26,\"margin\":15,\"minimumSpacing\":25,\"sides\":[{\"content\":{\"connectorIds\":[]},\"type\":\"ConnectorPlacement.EquallySpacedRectSide\",\"uuid\":\"f8ee33a9-954f-44c6-a821-b5353f3278fa\"},{\"content\":{\"connectorIds\":[],\"side\":\"RIGHT\"},\"type\":\"ConnectorPlacement.EquallySpacedRectSide\",\"uuid\":\"385f1e4f-1c89-4afc-9c19-76a078cf90bc\"},{\"content\":{\"connectorIds\":[],\"side\":\"TOP\"},\"type\":\"ConnectorPlacement.EquallySpacedRectSide\",\"uuid\":\"fc91fa49-46f5-4ba7-960e-7bda5e0416d1\"}]},\"type\":\"ConnectorPlacement.EquallySpacedConnector\",\"uuid\":\"4bf08bc6-c7ce-47fb-af04-cd9d2b5f8092\"}],\"packageUris\":[\"http://schema.mathworks.com/mf0/Connector/19700101\"],\"version\":\"1.0\"}"
  Wire 2 : Subsystem
      settings: PortSchema="{\"entries\":[{\"content\":{\"headerSize\":26,\"margin\":15,\"minimumSpacing\":25,\"sides\":[{\"content\":{\"connectorIds\":[]},\"type\":\"ConnectorPlacement.EquallySpacedRectSide\",\"uuid\":\"f8ee33a9-954f-44c6-a821-b5353f3278fa\"},{\"content\":{\"connectorIds\":[],\"side\":\"RIGHT\"},\"type\":\"ConnectorPlacement.EquallySpacedRectSide\",\"uuid\":\"385f1e4f-1c89-4afc-9c19-76a078cf90bc\"},{\"content\":{\"connectorIds\":[],\"side\":\"TOP\"},\"type\":\"ConnectorPlacement.EquallySpacedRectSide\",\"uuid\":\"fc91fa49-46f5-4ba7-960e-7bda5e0416d1\"}]},\"type\":\"ConnectorPlacement.EquallySpacedConnector\",\"uuid\":\"4bf08bc6-c7ce-47fb-af04-cd9d2b5f8092\"}],\"packageUris\":[\"http://schema.mathworks.com/mf0/Connector/19700101\"],\"version\":\"1.0\"}"
  Wire 3 : Subsystem
      settings: PortSchema="{\"entries\":[{\"content\":{\"headerSize\":26,\"margin\":15,\"minimumSpacing\":25,\"sides\":[{\"content\":{\"connectorIds\":[]},\"type\":\"ConnectorPlacement.EquallySpacedRectSide\",\"uuid\":\"f8ee33a9-954f-44c6-a821-b5353f3278fa\"},{\"content\":{\"connectorIds\":[],\"side\":\"RIGHT\"},\"type\":\"ConnectorPlacement.EquallySpacedRectSide\",\"uuid\":\"385f1e4f-1c89-4afc-9c19-76a078cf90bc\"},{\"content\":{\"connectorIds\":[],\"side\":\"TOP\"},\"type\":\"ConnectorPlacement.EquallySpacedRectSide\",\"uuid\":\"fc91fa49-46f5-4ba7-960e-7bda5e0416d1\"}]},\"type\":\"ConnectorPlacement.EquallySpacedConnector\",\"uuid\":\"4bf08bc6-c7ce-47fb-af04-cd9d2b5f8092\"}],\"packageUris\":[\"http://schema.mathworks.com/mf0/Connector/19700101\"],\"version\":\"1.0\"}"
  Wire 4 : Subsystem
      settings: PortSchema="{\"entries\":[{\"content\":{\"headerSize\":26,\"margin\":15,\"minimumSpacing\":25,\"sides\":[{\"content\":{\"connectorIds\":[]},\"type\":\"ConnectorPlacement.EquallySpacedRectSide\",\"uuid\":\"f8ee33a9-954f-44c6-a821-b5353f3278fa\"},{\"content\":{\"connectorIds\":[],\"side\":\"RIGHT\"},\"type\":\"ConnectorPlacement.EquallySpacedRectSide\",\"uuid\":\"385f1e4f-1c89-4afc-9c19-76a078cf90bc\"},{\"content\":{\"connectorIds\":[],\"side\":\"TOP\"},\"type\":\"ConnectorPlacement.EquallySpacedRectSide\",\"uuid\":\"fc91fa49-46f5-4ba7-960e-7bda5e0416d1\"}]},\"type\":\"ConnectorPlacement.EquallySpacedConnector\",\"uuid\":\"4bf08bc6-c7ce-47fb-af04-cd9d2b5f8092\"}],\"packageUris\":[\"http://schema.mathworks.com/mf0/Connector/19700101\"],\"version\":\"1.0\"}"
  Wire 5 : Subsystem
      settings: PortSchema="{\"entries\":[{\"content\":{\"headerSize\":26,\"margin\":15,\"minimumSpacing\":25,\"sides\":[{\"content\":{\"connectorIds\":[]},\"type\":\"ConnectorPlacement.EquallySpacedRectSide\",\"uuid\":\"f8ee33a9-954f-44c6-a821-b5353f3278fa\"},{\"content\":{\"connectorIds\":[],\"side\":\"RIGHT\"},\"type\":\"ConnectorPlacement.EquallySpacedRectSide\",\"uuid\":\"385f1e4f-1c89-4afc-9c19-76a078cf90bc\"},{\"content\":{\"connectorIds\":[],\"side\":\"TOP\"},\"type\":\"ConnectorPlacement.EquallySpacedRectSide\",\"uuid\":\"fc91fa49-46f5-4ba7-960e-7bda5e0416d1\"}]},\"type\":\"ConnectorPlacement.EquallySpacedConnector\",\"uuid\":\"4bf08bc6-c7ce-47fb-af04-cd9d2b5f8092\"}],\"packageUris\":[\"http://schema.mathworks.com/mf0/Connector/19700101\"],\"version\":\"1.0\"}"
  Wire 6 : Subsystem
      settings: PortSchema="{\"entries\":[{\"content\":{\"headerSize\":26,\"margin\":15,\"minimumSpacing\":25,\"sides\":[{\"content\":{\"connectorIds\":[]},\"type\":\"ConnectorPlacement.EquallySpacedRectSide\",\"uuid\":\"f8ee33a9-954f-44c6-a821-b5353f3278fa\"},{\"content\":{\"connectorIds\":[],\"side\":\"RIGHT\"},\"type\":\"ConnectorPlacement.EquallySpacedRectSide\",\"uuid\":\"385f1e4f-1c89-4afc-9c19-76a078cf90bc\"},{\"content\":{\"connectorIds\":[],\"side\":\"TOP\"},\"type\":\"ConnectorPlacement.EquallySpacedRectSide\",\"uuid\":\"fc91fa49-46f5-4ba7-960e-7bda5e0416d1\"}]},\"type\":\"ConnectorPlacement.EquallySpacedConnector\",\"uuid\":\"4bf08bc6-c7ce-47fb-af04-cd9d2b5f8092\"}],\"packageUris\":[\"http://schema.mathworks.com/mf0/Connector/19700101\"],\"version\":\"1.0\"}"

== system p4_system_arch_master/System 6 : Sensor and Actuation System/6.1 Sensor System /6.1.7 Motor Position Measurement Subsystem /6.1.7.2 Motor Resolver - Rotor Subsystem/6.1.7.2.1 Motor Resolver - Rotor Subsystem Body  ==

== system p4_system_arch_master/System 10 : Electrical Distribution System /10.2 LV Distribution System /10.2.1	Internal LV Loom System/10.2.1.1	Inverter to Motor LV loom system/PT100 #1 Wire System/10.2.1.1.18	PT100 #1 Wire "Ex+" ==

== system p4_system_arch_master/System 10 : Electrical Distribution System /10.2 LV Distribution System /10.2.1	Internal LV Loom System/10.2.1.1	Inverter to Motor LV loom system/PT100 #1 Wire System/10.2.1.1.19	PT100 #1 Wire "Ex-" ==

== system p4_system_arch_master/System 10 : Electrical Distribution System /10.2 LV Distribution System /10.2.1	Internal LV Loom System/10.2.1.1	Inverter to Motor LV loom system/PT100 #1 Wire System/10.2.1.1.20	PT100 #1 Wire "Ex+" Insulation ==

== system p4_system_arch_master/System 10 : Electrical Distribution System /10.2 LV Distribution System /10.2.1	Internal LV Loom System/10.2.1.1	Inverter to Motor LV loom system/PT100 #1 Wire System/10.2.1.1.21	PT100 #1 Wire "Ex-" Insulation ==

== system p4_system_arch_master/System 10 : Electrical Distribution System /10.2 LV Distribution System /10.2.1	Internal LV Loom System/10.2.1.1	Inverter to Motor LV loom system/PT100 #1 Wire System/10.2.1.1.22	PT100 #1 Wire pair "Ex" shielding braid ==

== system p4_system_arch_master/System 10 : Electrical Distribution System /10.2 LV Distribution System /10.2.1	Internal LV Loom System/10.2.1.1	Inverter to Motor LV loom system/PT100 #2 Wire System/10.2.1.1.23	PT100 #2 Wire "Ex+" ==

== system p4_system_arch_master/System 10 : Electrical Distribution System /10.2 LV Distribution System /10.2.1	Internal LV Loom System/10.2.1.1	Inverter to Motor LV loom system/PT100 #2 Wire System/10.2.1.1.24	PT100 #2 Wire "Ex-" ==

== system p4_system_arch_master/System 10 : Electrical Distribution System /10.2 LV Distribution System /10.2.1	Internal LV Loom System/10.2.1.1	Inverter to Motor LV loom system/PT100 #2 Wire System/10.2.1.1.25	PT100 #2 Wire "Ex+" Insulation ==

== system p4_system_arch_master/System 10 : Electrical Distribution System /10.2 LV Distribution System /10.2.1	Internal LV Loom System/10.2.1.1	Inverter to Motor LV loom system/PT100 #2 Wire System/10.2.1.1.26	PT100 #2 Wire "Ex-" Insulation ==

== system p4_system_arch_master/System 10 : Electrical Distribution System /10.2 LV Distribution System /10.2.1	Internal LV Loom System/10.2.1.1	Inverter to Motor LV loom system/PT100 #2 Wire System/10.2.1.1.27	PT100 #2 Wire pair "Ex" shielding braid ==

== system p4_system_arch_master/System 10 : Electrical Distribution System /10.2 LV Distribution System /10.2.1	Internal LV Loom System/10.2.1.1	Inverter to Motor LV loom system/Resolver sensor System/10.2.1.1.02	Resolver sensor connector ==

== system p4_system_arch_master/System 10 : Electrical Distribution System /10.2 LV Distribution System /10.2.1	Internal LV Loom System/10.2.1.1	Inverter to Motor LV loom system/Resolver sensor System/10.2.1.1.03	Resolver sensor  Wires ==
  10.2.1.1.08	Resolver sensor  Wire Cos : Subsystem
      settings: PortSchema="{\"entries\":[{\"content\":{\"headerSize\":26,\"margin\":15,\"minimumSpacing\":25,\"sides\":[{\"content\":{\"connectorIds\":[]},\"type\":\"ConnectorPlacement.EquallySpacedRectSide\",\"uuid\":\"f8ee33a9-954f-44c6-a821-b5353f3278fa\"},{\"content\":{\"connectorIds\":[],\"side\":\"RIGHT\"},\"type\":\"ConnectorPlacement.EquallySpacedRectSide\",\"uuid\":\"385f1e4f-1c89-4afc-9c19-76a078cf90bc\"},{\"content\":{\"connectorIds\":[],\"side\":\"TOP\"},\"type\":\"ConnectorPlacement.EquallySpacedRectSide\",\"uuid\":\"fc91fa49-46f5-4ba7-960e-7bda5e0416d1\"}]},\"type\":\"ConnectorPlacement.EquallySpacedConnector\",\"uuid\":\"4bf08bc6-c7ce-47fb-af04-cd9d2b5f8092\"}],\"packageUris\":[\"http://schema.mathworks.com/mf0/Connector/19700101\"],\"version\":\"1.0\"}"
  Resolver sensor  Wire Sin : Subsystem
      settings: PortSchema="{\"entries\":[{\"content\":{\"headerSize\":26,\"margin\":15,\"minimumSpacing\":25,\"sides\":[{\"content\":{\"connectorIds\":[]},\"type\":\"ConnectorPlacement.EquallySpacedRectSide\",\"uuid\":\"f8ee33a9-954f-44c6-a821-b5353f3278fa\"},{\"content\":{\"connectorIds\":[],\"side\":\"RIGHT\"},\"type\":\"ConnectorPlacement.EquallySpacedRectSide\",\"uuid\":\"385f1e4f-1c89-4afc-9c19-76a078cf90bc\"},{\"content\":{\"connectorIds\":[],\"side\":\"TOP\"},\"type\":\"ConnectorPlacement.EquallySpacedRectSide\",\"uuid\":\"fc91fa49-46f5-4ba7-960e-7bda5e0416d1\"}]},\"type\":\"ConnectorPlacement.EquallySpacedConnector\",\"uuid\":\"4bf08bc6-c7ce-47fb-af04-cd9d2b5f8092\"}],\"packageUris\":[\"http://schema.mathworks.com/mf0/Connector/19700101\"],\"version\":\"1.0\"}"
  Resolver sensor Wire Ex : Subsystem
      settings: PortSchema="{\"entries\":[{\"content\":{\"headerSize\":26,\"margin\":15,\"minimumSpacing\":25,\"sides\":[{\"content\":{\"connectorIds\":[]},\"type\":\"ConnectorPlacement.EquallySpacedRectSide\",\"uuid\":\"f8ee33a9-954f-44c6-a821-b5353f3278fa\"},{\"content\":{\"connectorIds\":[],\"side\":\"RIGHT\"},\"type\":\"ConnectorPlacement.EquallySpacedRectSide\",\"uuid\":\"385f1e4f-1c89-4afc-9c19-76a078cf90bc\"},{\"content\":{\"connectorIds\":[],\"side\":\"TOP\"},\"type\":\"ConnectorPlacement.EquallySpacedRectSide\",\"uuid\":\"fc91fa49-46f5-4ba7-960e-7bda5e0416d1\"}]},\"type\":\"ConnectorPlacement.EquallySpacedConnector\",\"uuid\":\"4bf08bc6-c7ce-47fb-af04-cd9d2b5f8092\"}],\"packageUris\":[\"http://schema.mathworks.com/mf0/Connector/19700101\"],\"version\":\"1.0\"}"

== system p4_system_arch_master/System 10 : Electrical Distribution System /10.2 LV Distribution System /10.2.1	Internal LV Loom System/10.2.1.2	Inverter to Inverter LV connector loom system/Inverter Internal Wires/CAN1_H Wire ==
  "10.2.1.2.06\tInverter internal wire \"CAN1_H\"" : Subsystem
      settings: PortSchema="{\"entries\":[{\"content\":{\"headerSize\":26,\"margin\":15,\"minimumSpacing\":25,\"sides\":[{\"content\":{\"connectorIds\":[]},\"type\":\"ConnectorPlacement.EquallySpacedRectSide\",\"uuid\":\"f8ee33a9-954f-44c6-a821-b5353f3278fa\"},{\"content\":{\"connectorIds\":[],\"side\":\"RIGHT\"},\"type\":\"ConnectorPlacement.EquallySpacedRectSide\",\"uuid\":\"385f1e4f-1c89-4afc-9c19-76a078cf90bc\"},{\"content\":{\"connectorIds\":[],\"side\":\"TOP\"},\"type\":\"ConnectorPlacement.EquallySpacedRectSide\",\"uuid\":\"fc91fa49-46f5-4ba7-960e-7bda5e0416d1\"}]},\"type\":\"ConnectorPlacement.EquallySpacedConnector\",\"uuid\":\"4bf08bc6-c7ce-47fb-af04-cd9d2b5f8092\"}],\"packageUris\":[\"http://schema.mathworks.com/mf0/Connector/19700101\"],\"version\":\"1.0\"}"
  "10.2.1.2.18\tInverter internal wire \"CAN1_H\" insulation" : Subsystem
      settings: PortSchema="{\"entries\":[{\"content\":{\"headerSize\":26,\"margin\":15,\"minimumSpacing\":25,\"sides\":[{\"content\":{\"connectorIds\":[]},\"type\":\"ConnectorPlacement.EquallySpacedRectSide\",\"uuid\":\"f8ee33a9-954f-44c6-a821-b5353f3278fa\"},{\"content\":{\"connectorIds\":[],\"side\":\"RIGHT\"},\"type\":\"ConnectorPlacement.EquallySpacedRectSide\",\"uuid\":\"385f1e4f-1c89-4afc-9c19-76a078cf90bc\"},{\"content\":{\"connectorIds\":[],\"side\":\"TOP\"},\"type\":\"ConnectorPlacement.EquallySpacedRectSide\",\"uuid\":\"fc91fa49-46f5-4ba7-960e-7bda5e0416d1\"}]},\"type\":\"ConnectorPlacement.EquallySpacedConnector\",\"uuid\":\"4bf08bc6-c7ce-47fb-af04-cd9d2b5f8092\"}],\"packageUris\":[\"http://schema.mathworks.com/mf0/Connector/19700101\"],\"version\":\"1.0\"}"

== system p4_system_arch_master/System 10 : Electrical Distribution System /10.2 LV Distribution System /10.2.1	Internal LV Loom System/10.2.1.2	Inverter to Inverter LV connector loom system/Inverter Internal Wires/CAN1_L Wire ==
  "10.2.1.2.12\tInverter internal wire \"CAN1_L\"" : Subsystem
      settings: PortSchema="{\"entries\":[{\"content\":{\"headerSize\":26,\"margin\":15,\"minimumSpacing\":25,\"sides\":[{\"content\":{\"connectorIds\":[]},\"type\":\"ConnectorPlacement.EquallySpacedRectSide\",\"uuid\":\"f8ee33a9-954f-44c6-a821-b5353f3278fa\"},{\"content\":{\"connectorIds\":[],\"side\":\"RIGHT\"},\"type\":\"ConnectorPlacement.EquallySpacedRectSide\",\"uuid\":\"385f1e4f-1c89-4afc-9c19-76a078cf90bc\"},{\"content\":{\"connectorIds\":[],\"side\":\"TOP\"},\"type\":\"ConnectorPlacement.EquallySpacedRectSide\",\"uuid\":\"fc91fa49-46f5-4ba7-960e-7bda5e0416d1\"}]},\"type\":\"ConnectorPlacement.EquallySpacedConnector\",\"uuid\":\"4bf08bc6-c7ce-47fb-af04-cd9d2b5f8092\"}],\"packageUris\":[\"http://schema.mathworks.com/mf0/Connector/19700101\"],\"version\":\"1.0\"}"
  "10.2.1.2.24\tInverter internal wire \"CAN1_L\" insulation" : Subsystem
      settings: PortSchema="{\"entries\":[{\"content\":{\"headerSize\":26,\"margin\":15,\"minimumSpacing\":25,\"sides\":[{\"content\":{\"connectorIds\":[]},\"type\":\"ConnectorPlacement.EquallySpacedRectSide\",\"uuid\":\"f8ee33a9-954f-44c6-a821-b5353f3278fa\"},{\"content\":{\"connectorIds\":[],\"side\":\"RIGHT\"},\"type\":\"ConnectorPlacement.EquallySpacedRectSide\",\"uuid\":\"385f1e4f-1c89-4afc-9c19-76a078cf90bc\"},{\"content\":{\"connectorIds\":[],\"side\":\"TOP\"},\"type\":\"ConnectorPlacement.EquallySpacedRectSide\",\"uuid\":\"fc91fa49-46f5-4ba7-960e-7bda5e0416d1\"}]},\"type\":\"ConnectorPlacement.EquallySpacedConnector\",\"uuid\":\"4bf08bc6-c7ce-47fb-af04-cd9d2b5f8092\"}],\"packageUris\":[\"http://schema.mathworks.com/mf0/Connector/19700101\"],\"version\":\"1.0\"}"

== system p4_system_arch_master/System 10 : Electrical Distribution System /10.2 LV Distribution System /10.2.1	Internal LV Loom System/10.2.1.2	Inverter to Inverter LV connector loom system/Inverter Internal Wires/CAN2_H Wire ==
  "10.2.1.2.07\tInverter internal wire \"CAN2_H\"" : Subsystem
      settings: PortSchema="{\"entries\":[{\"content\":{\"headerSize\":26,\"margin\":15,\"minimumSpacing\":25,\"sides\":[{\"content\":{\"connectorIds\":[]},\"type\":\"ConnectorPlacement.EquallySpacedRectSide\",\"uuid\":\"f8ee33a9-954f-44c6-a821-b5353f3278fa\"},{\"content\":{\"connectorIds\":[],\"side\":\"RIGHT\"},\"type\":\"ConnectorPlacement.EquallySpacedRectSide\",\"uuid\":\"385f1e4f-1c89-4afc-9c19-76a078cf90bc\"},{\"content\":{\"connectorIds\":[],\"side\":\"TOP\"},\"type\":\"ConnectorPlacement.EquallySpacedRectSide\",\"uuid\":\"fc91fa49-46f5-4ba7-960e-7bda5e0416d1\"}]},\"type\":\"ConnectorPlacement.EquallySpacedConnector\",\"uuid\":\"4bf08bc6-c7ce-47fb-af04-cd9d2b5f8092\"}],\"packageUris\":[\"http://schema.mathworks.com/mf0/Connector/19700101\"],\"version\":\"1.0\"}"
  "10.2.1.2.19\tInverter internal wire \"CAN2_H\" insulation" : Subsystem
      settings: PortSchema="{\"entries\":[{\"content\":{\"headerSize\":26,\"margin\":15,\"minimumSpacing\":25,\"sides\":[{\"content\":{\"connectorIds\":[]},\"type\":\"ConnectorPlacement.EquallySpacedRectSide\",\"uuid\":\"f8ee33a9-954f-44c6-a821-b5353f3278fa\"},{\"content\":{\"connectorIds\":[],\"side\":\"RIGHT\"},\"type\":\"ConnectorPlacement.EquallySpacedRectSide\",\"uuid\":\"385f1e4f-1c89-4afc-9c19-76a078cf90bc\"},{\"content\":{\"connectorIds\":[],\"side\":\"TOP\"},\"type\":\"ConnectorPlacement.EquallySpacedRectSide\",\"uuid\":\"fc91fa49-46f5-4ba7-960e-7bda5e0416d1\"}]},\"type\":\"ConnectorPlacement.EquallySpacedConnector\",\"uuid\":\"4bf08bc6-c7ce-47fb-af04-cd9d2b5f8092\"}],\"packageUris\":[\"http://schema.mathworks.com/mf0/Connector/19700101\"],\"version\":\"1.0\"}"
